simulink model "Demo1Vtue22_3"  (R2015a)
settings: Solver=ode45  StartTime=0.0  StopTime=inf  RelTol=1e-3
InitFcn:
  | Initilization_simulink
values from neighbouring files (symbols this model uses):
  field_x = sqrt(field_x_vec(1)^2 + field_x_vec(2)^2)    [CalibrateField.m]    (also in Config.mat = 12.1039066508)
  field_y = sqrt(field_y_vec(1)^2 + field_y_vec(2)^2)    [CalibrateField.m]    (also in Config.mat = 7.80292411046)
  items = [CR1;CR2;CR3;CR4]    [CalibrateField.m]    (also in Config.mat = [-6.20782769901  -3.78898920633; 6.05245909893  -4.012387933)
  ref = [4.14037710566  -4.49582588886  0; 4.11853559592  4.24885683451  0; -2.83708842359  -4.61422491343  0]    [Config.mat]
  referenceImage = imread('field.png')    [Initilization_simulink.m]
  thetaCamX = 43*pi/180    (= 0.750491578358)    [Initilization_simulink.m]    (also in debugging_refereeing.m = 1.01229096616)
  thetaCamY = 32*pi/180    (= 0.558505360638)    [Initilization_simulink.m]
undefined symbols (not defined in the file or in its folder): backim, drone1
libraries: visionsinks x2
settings Model: CovSFcnEnable=off  Creator=tzwijger  LastModifiedBy=tzwijger
settings DebuggingCC: SolverPrmCheckMsg=warning

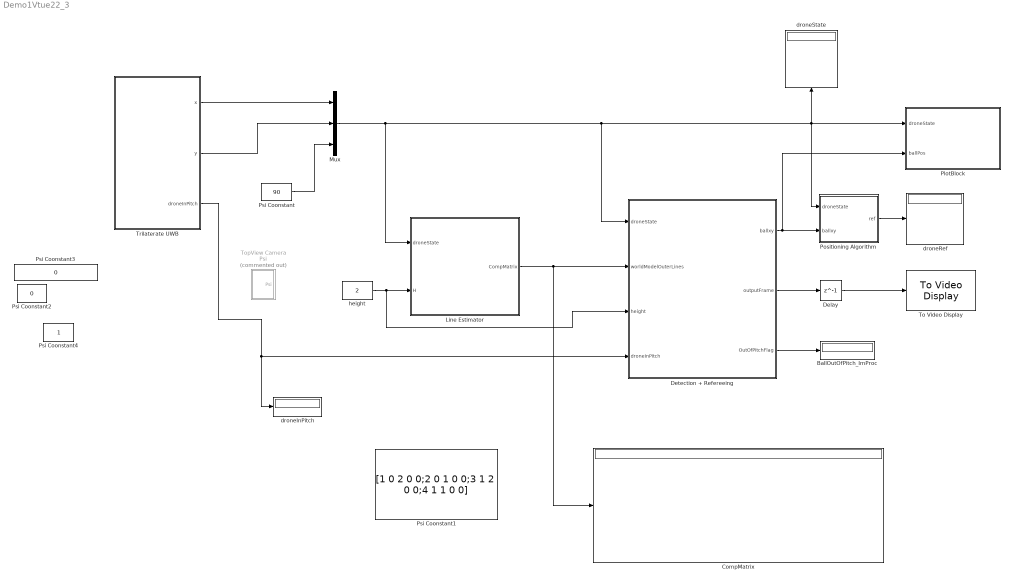
== system Demo1Vtue22_3 ==
  BallOutOfPitch_ImProc : Display
  CompMatrix : Display
  Delay : Delay  DelayLength=1  SampleTime=0.25
  Detection + Refereeing : Subsystem
  Line Estimator : Subsystem
  Mux : Mux  Inputs=3
  PlotBlock : Subsystem
  Positioning Algorithm : Subsystem
  Psi Coonstant : Constant  Value=90
  Psi Coonstant1 : Constant  Value=[1 0 2 0 0;2 0 1 0 0;3 1 2 0 0;4 1 1 0 0]
  Psi Coonstant2 : Constant  Value=0
  Psi Coonstant3 : Constant  Value=0
  Psi Coonstant4 : Constant
  To Video Display : visionsinks/To Video Display  windowSizeMode=True size (1:1)  openAtMdlStart=on  fullScreen=off  videoWindowX=1359  videoWindowY=403  saveWindowSize=off  videoWindowWidth=320  videoWindowHeight=240  inputColorFormat=RGB  inputType=Obsolete  imagePorts=One multidimensional signal  OutputDevice=On-screen video monitor  dataOrg=Column-major  isWindowOpen=off
  TopView Camera Psi : Subsystem  Commented=on
  Trilaterate UWB : Subsystem
  droneInPitch : Display
  droneRef : Display
  droneState : Display
  height : Constant  Value=2
  wires:
  Detection + Refereeing/3(OutOfPitchFlag) -> BallOutOfPitch_ImProc/1
  Line Estimator/1(CompMatrix) -> Detection + Refereeing/2(worldModelOuterLines), CompMatrix/1
  Trilaterate UWB/3(droneInPitch) -> droneInPitch/1, Detection + Refereeing/4(droneInPitch)
  height/1 -> Detection + Refereeing/3(height), Line Estimator/2(H)
  Mux/1 -> Line Estimator/1(droneState), Detection + Refereeing/1(droneState), PlotBlock/1(droneState), Positioning Algorithm/1(droneState), droneState/1
  Detection + Refereeing/1(ballxy) -> PlotBlock/2(ballPos), Positioning Algorithm/2(ballxy)
  Positioning Algorithm/1(ref) -> droneRef/1
  Psi Coonstant/1 -> Mux/3
  Detection + Refereeing/2(outputFrame) -> Delay/1
  Delay/1 -> To Video Display/1
  Trilaterate UWB/1(x) -> Mux/1
  Trilaterate UWB/2(y) -> Mux/2

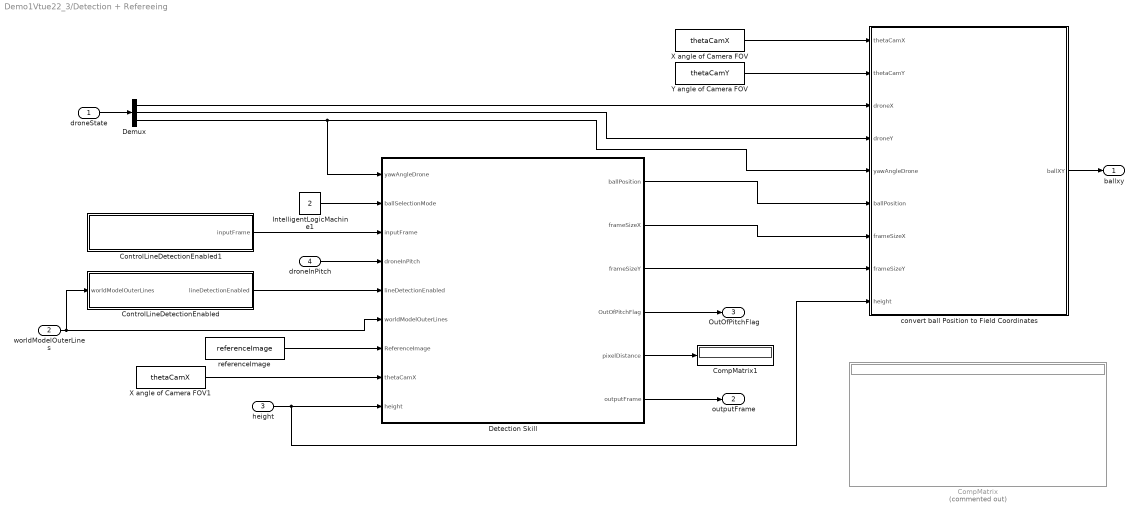
== system Demo1Vtue22_3/Detection + Refereeing ==
  droneState : Inport
  worldModelOuterLines : Inport  Port=2
  height : Inport  Port=3
  droneInPitch : Inport  Port=4
  CompMatrix : Display  Commented=on
  CompMatrix1 : Display
  ControlLineDetectionEnabled : MATLAB Function  TreatAsAtomicUnit=on
  ControlLineDetectionEnabled1 : MATLAB Function  TreatAsAtomicUnit=on
  Demux : Demux  Outputs=3
  Detection Skill : MATLAB Function  TreatAsAtomicUnit=on
  IntelligentLogicMachine1 : Constant  Value=2
  X angle of Camera FOV : Constant  Value=thetaCamX
  X angle of Camera FOV1 : Constant  Value=thetaCamX
  Y angle of Camera FOV : Constant  Value=thetaCamY
  convert ball Position to Field Coordinates : Subsystem
  referenceImage : Constant  Value=referenceImage
  ballxy : Outport
  outputFrame : Outport  Port=2
  OutOfPitchFlag : Outport  Port=3
  wires:
  worldModelOuterLines/1 -> Detection Skill/6(worldModelOuterLines), ControlLineDetectionEnabled/1(worldModelOuterLines)
  droneState/1 -> Demux/1
  Demux/3 -> Detection Skill/1(yawAngleDrone), convert ball Position to Field Coordinates/5(yawAngleDrone)
  Demux/1 -> convert ball Position to Field Coordinates/3(droneX)
  Demux/2 -> convert ball Position to Field Coordinates/4(droneY)
  convert ball Position to Field Coordinates/1(ballXY) -> ballxy/1
  X angle of Camera FOV/1 -> convert ball Position to Field Coordinates/1(thetaCamX)
  Y angle of Camera FOV/1 -> convert ball Position to Field Coordinates/2(thetaCamY)
  height/1 -> convert ball Position to Field Coordinates/9(height), Detection Skill/9(height)
  X angle of Camera FOV1/1 -> Detection Skill/8(thetaCamX)
  referenceImage/1 -> Detection Skill/7(ReferenceImage)
  ControlLineDetectionEnabled/1(lineDetectionEnabled) -> Detection Skill/5(lineDetectionEnabled)
  droneInPitch/1 -> Detection Skill/4(droneInPitch)
  ControlLineDetectionEnabled1/1(inputFrame) -> Detection Skill/3(inputFrame)
  IntelligentLogicMachine1/1 -> Detection Skill/2(ballSelectionMode)
  Detection Skill/5(pixelDistance) -> CompMatrix1/1
  Detection Skill/6(outputFrame) -> outputFrame/1
  Detection Skill/4(OutOfPitchFlag) -> OutOfPitchFlag/1
  Detection Skill/1(ballPosition) -> convert ball Position to Field Coordinates/6(ballPosition)
  Detection Skill/2(frameSizeX) -> convert ball Position to Field Coordinates/7(frameSizeX)
  Detection Skill/3(frameSizeY) -> convert ball Position to Field Coordinates/8(frameSizeY)

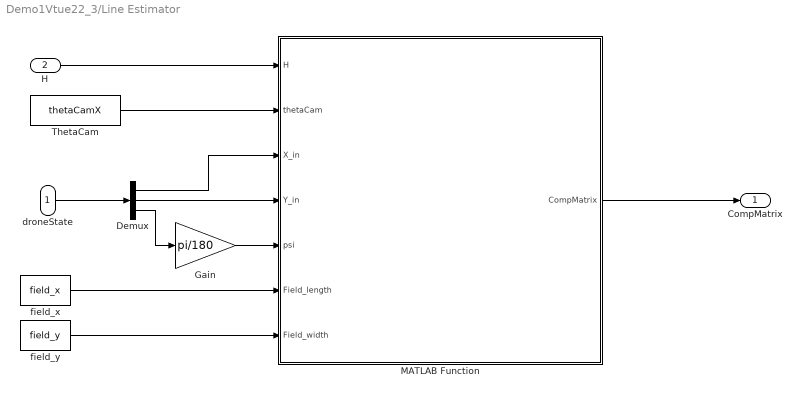
== system Demo1Vtue22_3/Line Estimator ==
  droneState : Inport
  H : Inport  Port=2
  Demux : Demux  Outputs=3
  Gain : Gain  Gain=pi/180
  MATLAB Function : MATLAB Function  TreatAsAtomicUnit=on
  ThetaCam : Constant  Value=thetaCamX
  field_x : Constant  Value=field_x
  field_y : Constant  Value=field_y
  CompMatrix : Outport
  wires:
  MATLAB Function/1(CompMatrix) -> CompMatrix/1
  ThetaCam/1 -> MATLAB Function/2(thetaCam)
  H/1 -> MATLAB Function/1(H)
  droneState/1 -> Demux/1
  field_x/1 -> MATLAB Function/6(Field_length)
  field_y/1 -> MATLAB Function/7(Field_width)
  Demux/1 -> MATLAB Function/3(X_in)
  Demux/2 -> MATLAB Function/4(Y_in)
  Demux/3 -> Gain/1
  Gain/1 -> MATLAB Function/5(psi)

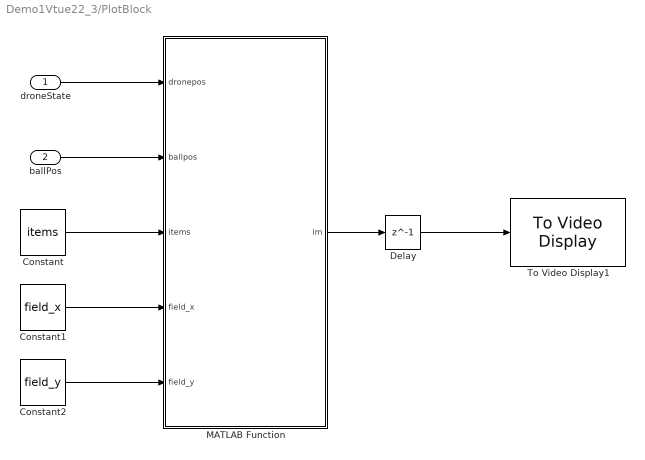
== system Demo1Vtue22_3/PlotBlock ==
  droneState : Inport
  ballPos : Inport  Port=2
  Constant : Constant  Value=items
  Constant1 : Constant  Value=field_x
  Constant2 : Constant  Value=field_y
  Delay : Delay  DelayLength=1  SampleTime=1
  MATLAB Function : MATLAB Function  TreatAsAtomicUnit=on
  To Video Display1 : visionsinks/To Video Display  windowSizeMode=True size (1:1)  openAtMdlStart=on  fullScreen=off  videoWindowX=992  videoWindowY=31  saveWindowSize=off  videoWindowWidth=810  videoWindowHeight=542  inputColorFormat=RGB  inputType=Obsolete  imagePorts=One multidimensional signal  OutputDevice=On-screen video monitor  dataOrg=Column-major  isWindowOpen=off
  wires:
  Constant/1 -> MATLAB Function/3(items)
  ballPos/1 -> MATLAB Function/2(ballpos)
  droneState/1 -> MATLAB Function/1(dronepos)
  Constant1/1 -> MATLAB Function/4(field_x)
  Constant2/1 -> MATLAB Function/5(field_y)
  MATLAB Function/1(im) -> Delay/1
  Delay/1 -> To Video Display1/1

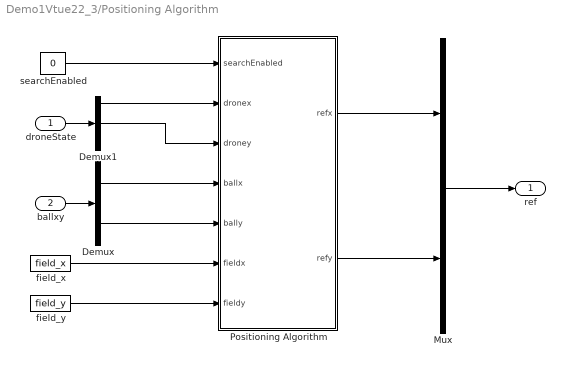
== system Demo1Vtue22_3/Positioning Algorithm ==
  droneState : Inport
  ballxy : Inport  Port=2
  Demux : Demux  Outputs=2
  Demux1 : Demux  Outputs=3
  Mux : Mux  Inputs=2
  Positioning Algorithm : MATLAB Function  TreatAsAtomicUnit=on
  field_x : Constant  Value=field_x
  field_y : Constant  Value=field_y
  searchEnabled : Constant  Value=0
  ref : Outport
  wires:
  Demux/2 -> Positioning Algorithm/5(bally)
  Demux/1 -> Positioning Algorithm/4(ballx)
  Positioning Algorithm/1(refx) -> Mux/1
  Positioning Algorithm/2(refy) -> Mux/2
  Mux/1 -> ref/1
  field_x/1 -> Positioning Algorithm/6(fieldx)
  field_y/1 -> Positioning Algorithm/7(fieldy)
  droneState/1 -> Demux1/1
  Demux1/1 -> Positioning Algorithm/2(dronex)
  ballxy/1 -> Demux/1
  Demux1/2 -> Positioning Algorithm/3(droney)
  searchEnabled/1 -> Positioning Algorithm/1(searchEnabled)

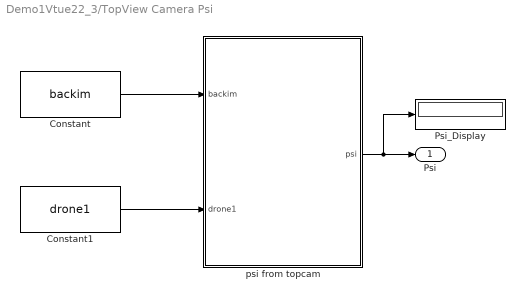
== system Demo1Vtue22_3/TopView Camera Psi ==
  Constant : Constant  Value=backim
  Constant1 : Constant  Value=drone1
  Psi_Display : Display
  psi from topcam : MATLAB Function  TreatAsAtomicUnit=on
  Psi : Outport
  wires:
  Constant1/1 -> psi from topcam/2(drone1)
  Constant/1 -> psi from topcam/1(backim)
  psi from topcam/1(psi) -> Psi_Display/1, Psi/1

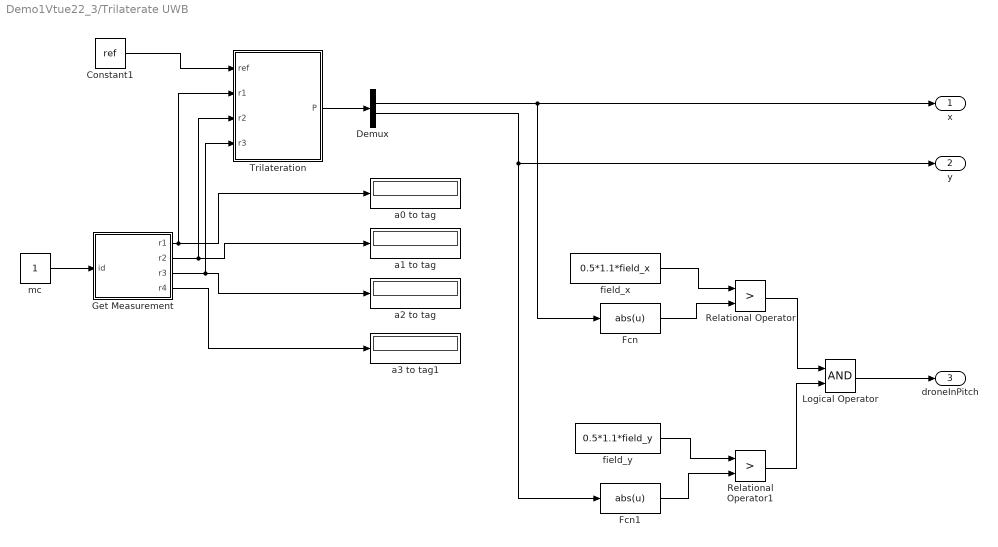
== system Demo1Vtue22_3/Trilaterate UWB ==
  Constant1 : Constant  Value=ref
  Demux : Demux
  Fcn : Fcn  Expr=abs(u)
  Fcn1 : Fcn  Expr=abs(u)
  Get Measurement : MATLAB Function  TreatAsAtomicUnit=on
  Logical Operator : Logic  AllPortsSameDT=off  OutDataTypeStr=boolean
  Relational Operator : RelationalOperator  Operator=>  OutDataTypeStr=boolean
  Relational Operator1 : RelationalOperator  Operator=>  OutDataTypeStr=boolean
  Trilateration : MATLAB Function  TreatAsAtomicUnit=on
  a0 to tag : Display
  a1 to tag : Display
  a2 to tag : Display
  a3 to tag1 : Display
  field_x : Constant  Value=0.5*1.1*field_x
  field_y : Constant  Value=0.5*1.1*field_y
  mc : Constant
  x : Outport
  y : Outport  Port=2
  droneInPitch : Outport  Port=3
  wires:
  Demux/3 -> Fcn1/1, y/1
  Demux/2 -> Fcn/1, x/1
  Trilateration/1(P) -> Demux/1
  Constant1/1 -> Trilateration/1(ref)
  Get Measurement/3(r3) -> a2 to tag/1, Trilateration/4(r3)
  Get Measurement/2(r2) -> a1 to tag/1, Trilateration/3(r2)
  mc/1 -> Get Measurement/1(id)
  Get Measurement/1(r1) -> Trilateration/2(r1), a0 to tag/1
  Get Measurement/4(r4) -> a3 to tag1/1
  Fcn/1 -> Relational Operator/2
  field_x/1 -> Relational Operator/1
  field_y/1 -> Relational Operator1/1
  Fcn1/1 -> Relational Operator1/2
  Relational Operator1/1 -> Logical Operator/2
  Relational Operator/1 -> Logical Operator/1
  Logical Operator/1 -> droneInPitch/1

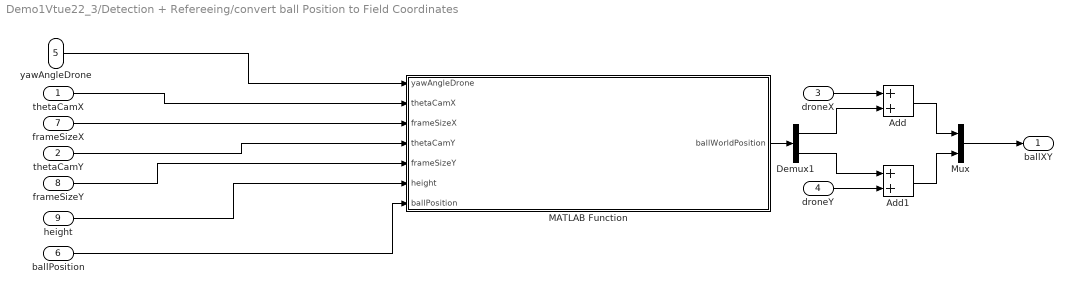
== system Demo1Vtue22_3/Detection + Refereeing/convert ball Position to Field Coordinates ==
  thetaCamX : Inport
  thetaCamY : Inport  Port=2
  droneX : Inport  Port=3
  droneY : Inport  Port=4
  yawAngleDrone : Inport  Port=5
  ballPosition : Inport  Port=6
  frameSizeX : Inport  Port=7
  frameSizeY : Inport  Port=8
  height : Inport  Port=9
  Add : Sum
  Add1 : Sum
  Demux1 : Demux  Outputs=2
  MATLAB Function : MATLAB Function  TreatAsAtomicUnit=on
  Mux : Mux  Inputs=2
  ballXY : Outport
  wires:
  thetaCamY/1 -> MATLAB Function/4(thetaCamY)
  height/1 -> MATLAB Function/6(height)
  yawAngleDrone/1 -> MATLAB Function/1(yawAngleDrone)
  thetaCamX/1 -> MATLAB Function/2(thetaCamX)
  ballPosition/1 -> MATLAB Function/7(ballPosition)
  frameSizeY/1 -> MATLAB Function/5(frameSizeY)
  Mux/1 -> ballXY/1
  Add/1 -> Mux/1
  Add1/1 -> Mux/2
  MATLAB Function/1(ballWorldPosition) -> Demux1/1
  frameSizeX/1 -> MATLAB Function/3(frameSizeX)
  droneX/1 -> Add/1
  Demux1/2 -> Add1/1
  Demux1/1 -> Add/2
  droneY/1 -> Add1/2

== matlab function Demo1Vtue22_3/Trilaterate UWB/Trilateration ==
  data: P output; ref input; r1 input; r2 input; r3 input
function P  = trilateration(ref,r1,r2,r3)%,fign,field2im_params)
% persistent plots k nrplots

coder.extrinsic('Trilateration')

% if isempty(plots)
%     plots = [0];
%     k = 1;
%     nrplots = 10;
% end

P = zeros(4,1);
P = Trilateration(ref',[r1 r2 r3],eye(3));

% % Plot and print results
% [plots, k] = update_plot_trilat(plots, k, fign, P(2:3), field2im_params, nrplots);

== matlab function Demo1Vtue22_3/Trilaterate UWB/Get Measurement ==
  data: id input; r1 output; r2 output; r3 output; r4 output
function [r1,r2,r3,r4] = GetMC_sm(id) 
    % Input: Serial Port to A0
    %        
    % Output: Raw data for triangulation
    %
    % Message syntax is explained in the Decawave documentation
    % DecaRangeRTLS_PC_Source_Code_Guide.pdf  - Section 2.3.2
    % DecaRangeRTLS_ARM_Source_Code_Guide.pdf - Section 2.6

    % Make sure to get a measurement with the correct identifier
    persistent s;
    %coder.extrinsic('instrfind','delete','serial','fscanf','strsplit')
    coder.extrinsic('instrfind','delete','serial','fscanf','GetMC')
    
    r1 = 0; r2 = 0; r3 = 0; r4 = 0;
    
    if isempty(s)
        ports = instrfind;
        if ~isempty(ports)
            fclose(ports);
            delete(ports);
        end
        % Establish new connection
        s = serial('COM33','BaudRate',9600,'Parity','None');

        % Open connection
        fopen(s);
        fscanf(s); % Get init mc out of the way and test connection
    end
    
    ids = ['mc';'mr';'ma'];
    id = ids(id,:);
    
    dist = zeros(1,4);
    dist = GetMC(s,id);
    r1 = dist(1);
    r2 = dist(2);
    r3 = dist(3);
    r4 = dist(4); 
end

== matlab function Demo1Vtue22_3/Line Estimator/MATLAB Function ==
  data: H input; CompMatrix output; thetaCam input; X_in input; Y_in input; psi input; Field_length input; Field_width input
function CompMatrix   = World(H,thetaCam,X_in,Y_in,psi,Field_length,Field_width)

% %field line numbering:  222222222222222222223
%                         1                   3
%                         1                   3
%                         1                   3
%                         1                   3
%                         1                   3
%                         144444444444444444443

% Psi: conter-clock wise positive. zero at localization Y axis
% Theta and rho are defined according to matlab hough transform matrix

Vision=2*H*tan(thetaCam/2);
X_Vision=Vision;  %<--------------->
Y_Vision=Vision*(480/640);  %|
                            %|
Lvision=sqrt((X_Vision^2)+(Y_Vision^2));
init_angel=atan(640/480);
X=X_in-(Lvision/2)*sin(init_angel-psi);  %moving the origin from center of the camera to top left
Y=Y_in+(Lvision/2)*cos(init_angel-psi);
%%%%%%%%%%%%%%%%%%%%%%%%%%%%%%%%%%%%%%%%%%%%%%%%%%%%%%%%%%%%%%%%%%%%%%%%%%
%Field_length=10;   %dimentions of the field%<--------------->

%Field_width=8; %|
                %|

%%%%%%%%%%%%%%%%%%%%%%%%%%%%%%%%%%%%%%%%%%%%%%%%%%%%%%%%%%%%%%%%%%%%%%%%%%%
rho1=abs(X+(Field_length)/2); %calculate rho of each side line with respect to top left cordinate
rho2=abs(-Y+(Field_width)/2);
rho3= abs(-X+(Field_length)/2);
rho4= abs(Y+(Field_width)/2);
%%%%%%%%%%%%%%%%%%%%%%%%%%%%%%%%%%%%%%%%%%%%%%%%%%%%%%%%%%%%%%%%%%%%%%%%
X1=X_in;  %having center to compare the distance and rho
Y1=Y_in;

rho11=abs(X1+(Field_length)/2);
rho21=abs(-Y1+(Field_width)/2);
rho31= abs(-X1+(Field_length)/2);
rho41= abs(Y1+(Field_width)/2);



%%%%%%%%%%%%%%%%%%%%%%%%%%%%%%%%%%%%%%%%%%%%%%%%%%%%%%%%%%%%%%%%%%%%%%%%%%
theta1=(pi)-psi;       %calculate the theta of each side line
theta2=(-pi/2)-psi;
theta3=(0)-psi;
theta4=(pi/2)-psi;
%%%%%%%%%%%%%%%%%%%%%%%%%%%%%%%%%%%%%%%%%%%%%%%%%%%%%%%%%%%%%%%%%%%%%%%%%%

Lines=[rho1,theta1,rho11;
rho2,theta2,rho21;
rho3,theta3,rho31;
rho4,theta4,rho41];
B=zeros(4,5);



for k=1:4
    
    i=0;
    rho=Lines(k,1);
    theta=Lines(k,2);
    %if -Y_Vision*sin(theta)<rho &&  rho<X_Vision*cos(theta)
    if Lines(k,3)<X_Vision/2
        i=1;
        

    end
    while theta>=(2*pi) 
        theta=theta-2*pi;
    end
    while theta<0
        theta=theta+2*pi;
    end
    
        while theta>=(pi/2) 
        theta=theta-pi;
    end
    while theta<-pi/2
        theta=theta+pi;
    end
    
    B(k,:)=[k i 0 rho theta];
end
B(1,3)=2;
B(2,3)=1;
B(3,3)=2;
B(4,3)=1;

CompMatrix=B;

== matlab function Demo1Vtue22_3/Detection + Refereeing/Detection Skill ==
  data: yawAngleDrone input; ballSelectionMode input; inputFrame input; droneInPitch input; lineDetectionEnabled input; worldModelOuterLines input; ReferenceImage input; thetaCamX input; height input; ballPosition output; frameSizeX output; frameSizeY output; OutOfPitchFlag output; pixelDistance output; outputFrame output
% Author: Nestor Hernandez Rodriguez
% Last Update: 9-03-2016
% Technical University of Eindhoven
% Mechatronic Systems Design PDEng trainee

function [ballPosition,...
          frameSizeX,...
          frameSizeY,...
          OutOfPitchFlag,...
          pixelDistance,...
          outputFrame] = detectionSkillAndRefereeing(...
                                                    yawAngleDrone,...
                                                    ballSelectionMode,... 
                                                    inputFrame,...
                                                    droneInPitch,...
                                                    lineDetectionEnabled,...
                                                    worldModelOuterLines,...
                                                    ReferenceImage,...
                                                    thetaCamX,...
                                                    height)
                                                 
    coder.extrinsic('detectionSkill','refereeingOutOfPitch','imresize')
    
    % Prepare outputs detection skill
    ballPosition = zeros(1,2);
    %selectedLines = zeros(50,2);
    ballStatusFlag = 0;
    lineStatusFlag = 0;
    %inputFrame = imresize(inputFrame,0.65,'bilinear');
    
    outputFrame = uint8(zeros(size(inputFrame)));
    
    % Prepare outputs Refereeing function
    OutOfPitchFlag = 0;
%     selectedFilteredLines = zeros(2,6);
    pixelDistance=0;
    
    % Prepare constant/unused inputs Refereeing function
    lineWidth = 0;
    numOutOfBoundLines = 0;
    numOutOfBoundLines = sum(worldModelOuterLines(:,2));
    
    % Prepare Other Outputs
    temp = size(inputFrame);
    frameSizeX = temp(2);
    frameSizeY = temp(1);
    frameProperties = [frameSizeY frameSizeX];
    
    [ballPosition,... 
     selectedLines,... 
     outputFrame] = detectionSkill(ballSelectionMode,... 
                                   lineDetectionEnabled,...
                                   ReferenceImage,...
                                   inputFrame);
                               
    selectedLines                                                             
    [OutOfPitchFlag,...
        pixelDistance]= refereeingOutOfPitch(yawAngleDrone,...
                                           ballPosition,...
                                           lineWidth,...
                                           selectedLines,...
                                           numOutOfBoundLines,...
                                           frameProperties,...
                                           droneInPitch,...
                                           thetaCamX,...
                                           height,...                                           
                                           worldModelOuterLines);
end

== matlab function Demo1Vtue22_3/TopView Camera Psi/psi from topcam ==
  data: backim input; psi output; drone1 input
function psi = fcn(backim, drone1)
%% get psi angle from top camera
% this function is the improcdrones.m implemented for ONLY ONE DRONE and 
% therefore reduced.




coder.extrinsic('psi_topviewcam_wrapped')
    
    psi = 0;
    psi = psi_topviewcam_wrapped(backim, drone1);

end

== matlab function Demo1Vtue22_3/Detection + Refereeing/ControlLineDetectionEnabled ==
  data: worldModelOuterLines input; lineDetectionEnabled output
function lineDetectionEnabled = ctrl_LineDetectionEnabled(worldModelOuterLines)
    if sum(worldModelOuterLines(:,2)) > 0
        lineDetectionEnabled = 1;
    else
        lineDetectionEnabled = 0; 
    end
    %lineDetectionEnabled = 0;
end

== matlab function Demo1Vtue22_3/Positioning Algorithm/Positioning Algorithm ==
  data: searchEnabled input; dronex input; droney input; ballx input; refx output; bally input; refy output; fieldx input; fieldy input
function [refx,refy] = positionDrone(searchEnabled,dronex,droney,ballx,bally,fieldx,fieldy)
% ball position [-999 -999] -> No Ball Position Known
    persistent searchArray count step
    if isempty(searchArray)
       count = 1;
       i = 1;
       step = 1;
       searchArray = zeros(100,2);% Size HAS to be predetermined (...Simulink...)
       for y = -0.5*fieldy:step:0.5*fieldy
          searchArray(i,:) =  [-0.5*fieldx,y];
          searchArray(i+1,:) =  [0.5*fieldx,y];
          i = i + 2;
       end
    end
    refx = 0;
    refy = 0;

    if ballx ~= -999 && bally ~= -999
        % Ball Position is known
        if abs(ballx) < 0.5*fieldx && abs(bally) < 0.5*fieldy
            % Ball is in field
            refx = ballx; 
            refy = bally;
        else
            % Ball is out of field
            % Go as close as possible without leaving the field
            refx = sign(ballx)*min(abs(ballx),0.5*fieldx);
            refy = sign(bally)*min(abs(bally),0.5*fieldy);       
        end
        % Reset count if search was enabled
        if count ~= 1
            count = 1;
        end
    elseif searchEnabled
        % Ball position is not known, search sequence initiated
        if (abs(dronex) - searchArray(count,1) < 0.25 ||...
            abs(droney) - searchArray(count,2) < 0.25)
            if count < 2*floor(fieldy/step)
                count = count + 1;
            else
                count = 1;
            end
        end
        refx = searchArray(count,1);
        refy = searchArray(count,2);
    else
        % Search disabled, hover over origin
        refx = 0;
        refy = 0;
    end

== matlab function Demo1Vtue22_3/Detection + Refereeing/convert ball Position to Field Coordinates/MATLAB Function ==
  data: yawAngleDrone input; thetaCamX input; frameSizeX input; thetaCamY input; frameSizeY input; height input; ballPosition input; ballWorldPosition output
% Author: Nestor Hernandez Rodriguez
% Last Update: 15-03-2016
% Technical University of Eindhoven
% Mechatronic Systems Design PDEng trainee

function ballWorldPosition =frameToWorldCoordinates(yawAngleDrone, thetaCamX, frameSizeX, thetaCamY, frameSizeY, height, ballPosition)

% This function carries out the ball position conversion from pixel frame
% coordinates to world model coordinates in meters
% 
% Inputs:
% ballPosition - 2x1 vector containing the center of the ball in the frame
%
% yawAngleDrone - yaw angle of the drone referenced to the world model coordinate system in radians
%
% thetaCamX, thetaCamY - angle in radians of the FOV of the camera used for both axis
%
% frameSizeX, frameSizeY - resolution in pixels for both axis
% 
% height - height of the drone in meters
%
% Outputs:
% ballWorldPosition - 2x1 vector containing the center of the ball in the
% frame referenced to the world model coordinate system orientation in
% meters



% Calculate Rotation matrix between the frame reference system and the
% world reference system
if ballPosition(1) == -100 && ballPosition(2) == -100
    ballWorldPosition = [-999 -999];
else    
    %syms t;

    %x_Rot = [1 0 0; 0 cos(t) -sin(t); 0 sin(t) cos(t)];
    %z_Rot = [cos(t) -sin(t) 0; sin(t) cos(t) 0; 0 0 1];

    Rx=rotx(-180);%eval(subs(x_Rot, t, -pi));
    Rz=rotz(yawAngleDrone*180/pi);%eval(subs(z_Rot, t, yawAngleDrone));


    % Calculate ball position with respect to the center of the frame

    ballPosition2=[ballPosition(1)-frameSizeX/2; ballPosition(2)-frameSizeY/2; 0];

    % Calculate vector in the local reference system with the same orientation
    % as the absolute reference system

    ballPosition3=Rx*Rz*ballPosition2;

    % Translate pixel distance into meters for both axis (Using two thetas is
    % more accurate)

    pixelDistanceX = (height*tan(thetaCamX/2))/(frameSizeX/2);
    pixelDistanceY = (height*tan(thetaCamY/2))/(frameSizeY/2);

    % Calculating ball position in meters

    ballWorldPosition=[ballPosition3(1)*pixelDistanceX ballPosition3(2)*pixelDistanceY];
end

== matlab function Demo1Vtue22_3/Detection + Refereeing/ControlLineDetectionEnabled1 ==
  data: inputFrame output
function inputFrame = rasPiCam()    	
    coder.extrinsic('getFramePi')

    inputFrame = uint8(zeros(240,320,3));
    inputFrame = getFramePi();
end

== matlab function Demo1Vtue22_3/PlotBlock/MATLAB Function ==
  data: dronepos input; im output; ballpos input; items input; field_x input; field_y input
function im  = update_plot_trilat(dronepos, ballpos, items,field_x,field_y)
    
    persistent im_init field2im_params
    
    coder.extrinsic('init_plot_trilat_img','update_plot_trilat_img')    
        
    if (isempty(im_init)||isempty(field2im_params))
        [im_init,field2im_params] = init_plot_trilat_img(items,field_x,field_y);        
    end
    
    im = uint8(zeros(542,810,3));
    im = update_plot_trilat_img(im_init,field2im_params,ballpos,dronepos);   
end
